simulink model "DirectedEvent6_2018a"  (R2018a)
settings: Solver=VariableStepAuto  StartTime=0.0  StopTime=0.1  RelTol=1e-3
settings Model: Creator=86188  LastModifiedBy=bzhan

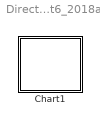
== system DirectedEvent6_2018a ==
  Chart1 : Stateflow chart  TreatAsAtomicUnit=on

== stateflow chart DirectedEvent6_2018a/Chart1 ==
  settings: updateMethod=DISCRETE  sampleTime=0.1
  state A
  state B
  state C
    state C1
    state C2
    (default) -> C1
    C1 -> C2 : F{f("d")}
  (default) -> A
  A -> B [order 1] : [data==1]{data=2;f("a");send(F,A);f("b")}
  A -> C [order 2] : F{f("c")}
  data: s function_input; data local =1
  events: F local FUNCTION_CALL_EVENT
  function f(s):
    | function f(s)
    |   fprintf(s+"\n");
